simulink model "halfband"  (Simulink 6.6)
settings: Solver=VariableStepDiscrete  SolverMode=SingleTasking  StartTime=0.0  StopTime=32768/12.8e6  RelTol=1e-3
PreLoadFcn:
  | BandStop = [-3.42958342739925E-03
  | -3.96924972816777E-03
  | 3.36240242079605E-03
  | -3.69559301938797E-04
  | -1.05894149003527E-03
  | -8.14840987107909E-04
  | 1.7530676387556E-03
  | 1.34036064966413E-04
  | -1.14308266128403E-03
  | -9.49174097090283E-05
  | 6.03248952668495E-04
  | -1.37880491661181E-05
  | 3.01496212854443E-04
  | -1.51170938115043E-04
  | -1.36598686838681E-03
  | 5.70111740975978E-04
  | 2.54687450879208E-03
  | -1.30938351650158E-03
  | -3.70345932594267E-03
  | 2.34958094527142E-03
  | 4.70638508861354E-03
  | -3.63447325770534E-03
  | -5.42048880850211E-03
  | 5.04733658994141E-03
  | 5.73664963492967E-03
  | -6.41806248410625E-03
  | -5.59266496429819E-03
  | 7.54327536806022E-03
  | 4.98552853346454E-03
  | -8.19477711532235E-03
  | -0.003981934398949
  | 8.15112472755439E-03
  | 2.73310679605007E-03
  | -7.2335178325926E-03
  | -1.46109700227312E-03
  | 5.31968276105546E-03
  | 4.53554392900545E-04
  | -2.3624905104136E-03
  | -6.91383416719793E-06
  | -1.55028072571844E-03
  | 4.39442000874746E-04
  | 6.24871824720405E-03
  | -2.02046112670604E-03
  | -1.14453241392008E-02
  | 4.95112589832473E-03
  | 1.67661124768428E-02
  | -9.32507740199684E-03
  | -0.021782122503324
  | 1.51131098154502E-02
  | 2.60432898181234E-02
  | -2.21466012963762E-02
  | -2.91212142686167E-02
  | 3.01168095402658E-02
  | 3.06633074260529E-02
  | -3.86045681695146E-02
  | -3.04226536102195E-02
  | 4.71064979395918E-02
  | 2.82864592477587E-02
  | -0.055072115030369
  | -2.43008385443716E-02
  | 6.19536218373718E-02
  | 1.86731297334143E-02
  | -6.72663181480251E-02
  | -1.17570405164474E-02
  | 7.06188933644473E-02
  | 4.01415550094957E-03
  | 0.928234958756191
  | 4.01415550094957E-03
  | 7.06188933644473E-02
  | -1.17570405164474E-02
  | -6.72663181480251E-02
  | 1.86731297334143E-02
  | 6.19536218373718E-02
  | -2.43008385443716E-02
  | -0.055072115030369
  | 2.82864592477587E-02
  | 4.71064979395918E-02
  | -3.04226536102195E-02
  | -3.86045681695146E-02
  | 3.06633074260529E-02
  | 3.01168095402658E-02
  | -2.91212142686167E-02
  | -2.21466012963762E-02
  | 2.60432898181234E-02
  | 1.51131098154502E-02
  | -0.021782122503324
  | -9.32507740199684E-03
  | 1.67661124768428E-02
  | 4.95112589832473E-03
  | -1.14453241392008E-02
  | -2.02046112670604E-03
  | 6.24871824720405E-03
  | 4.39442000874746E-04
  | -1.55028072571844E-03
  | -6.91383416719793E-06
  | -2.3624905104136E-03
  | 4.53554392900545E-04
  | 5.31968276105546E-03
  | -1.46109700227312E-03
  | -7.2335178325926E-03
  | 2.73310679605007E-03
  | 8.15112472755439E-03
  | -0.003981934398949
  | -8.19477711532235E-03
  | 4.98552853346454E-03
  | 7.54327536806022E-03
  | -5.59266496429819E-03
  | -6.41806248410625E-03
  | 5.73664963492967E-03
  | 5.04733658994141E-03
  | -5.42048880850211E-03
  | -3.63447325770534E-03
  | 4.70638508861354E-03
  | 2.34958094527142E-03
  | -3.70345932594267E-03
  | -1.30938351650158E-03
  | 2.54687450879208E-03
  | 5.70111740975978E-04
  | -1.36598686838681E-03
  | -1.51170938115043E-04
  | 3.01496212854443E-04
  | -1.37880491661181E-05
  | 6.03248952668495E-04
  | -9.49174097090283E-05
  | -1.14308266128403E-03
  | 1.34036064966413E-04
  | 1.7530676387556E-03
  | -8.14840987107909E-04
  | -1.05894149003527E-03
  | -3.69559301938797E-04
  | 3.36240242079605E-03
  | -3.96924972816777E-03
  | -3.42958342739925E-03];
undefined symbols (not defined in the file): dfilt
libraries: xbsIndex_r4 x78, dsparch4 x3, dspsigops x2
(part 1 of 2)
settings Model: Creator=lcrockett  LastModifiedBy=Administrator
settings DataIOCC: SignalLoggingName=sigsOut
settings OptimizationCC: InlineParams=on
settings DebuggingCC: SignalResolutionControl=TryResolveAllWithWarning  SolverPrmCheckMsg=none  MultiTaskDSMMsg=warning  MultiTaskCondExecSysMsg=none  StrictBusMsg=None
settings HardwareCC: TargetUnknown=on
settings RTWCC: IncludeERTFirstTime=on
settings GRTTargetCC: ModelReferenceCompliant=off  MatFileLogging=off

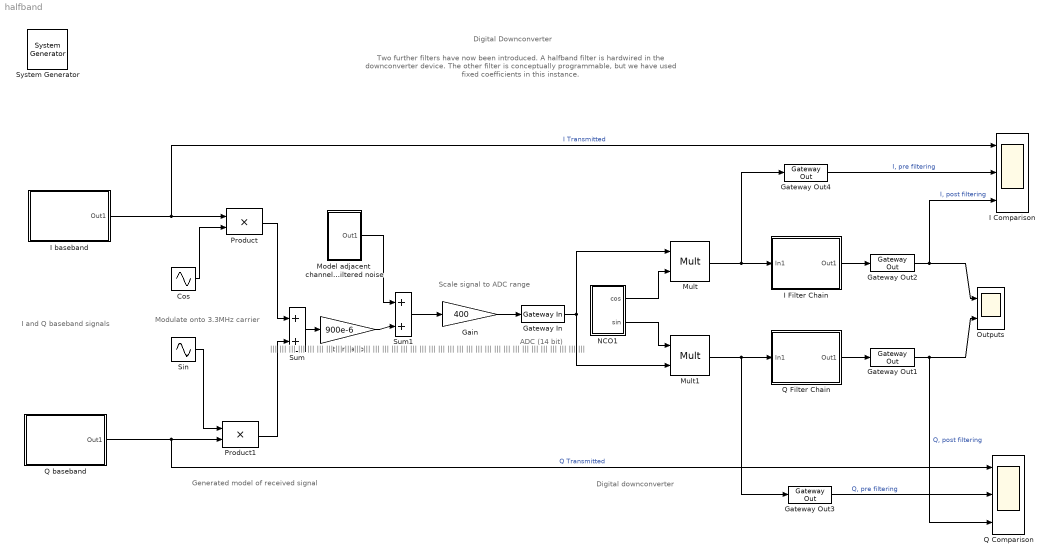
== system halfband ==
  note: Digital Downconverter
  note: Two further filters have now been introduced. A halfband filter is hardwired in the downconverter device.
      | The other filter is conceptually programmable, but we have used fixed coefficients in this instance.
  note: Digital downconverter
  note: ADC (14 bit)
  note: I and Q
      | baseband
      | signals
  note: Modulate onto
      | 3.3MHz carrier
  note: |||
      | |||
      | |||
      | |||
      | |||
      | |||
      | |||
      | |||
      | |||
      | |||
      | |||
      | |||
      | |||
      | |||
      | |||
      | |||
      | |||
      | |||
      | |||
      | |||
      | |||
      | |||
      | |||
      | |||
      | |||
      | |||
      | |||
      | |||
      | |||
      | |||
      | |||
      | |||
      | |||
      | |||
  note: Generated model of received signal
  note: Scale signal
      | to ADC range
  " System Generator" : xbsIndex_r4/ System Generator  Tag=genX  SystemSampleTime=-1  xilinxfamily=virtex2p  part=xc2vp30  speed=-7  package=ff896  synthesis_tool=XST  clock_wrapper=Clock Enables  directory=./netlist_05  testbench=off  simulink_period=1/12.8e6  sysclk_period=78.125  dcm_input_clock_period=100  incr_netlist=off  trim_vbits=Everywhere in SubSystem  dbl_ovrd=According to Block Masks  core_generation=According to Block Masks  run_coregen=off  deprecated_control=off  eval_field=0  block_type=sysgen
      settings: block_version=9.2.01
  Attenuation : Gain  Gain=900e-6  SaturateOnIntegerOverflow=on
  Cos : Sin  Frequency=2*pi*3.30999970436096e6  Phase=pi/2  SampleTime=1/12.8e6
  Gain : Gain  Gain=400  SaturateOnIntegerOverflow=on
  Gateway In : xbsIndex_r4/Gateway In  arith_type="Signed  (2's comp)"  n_bits=14  bin_pt=13  quantization="Round  (unbiased: +/- Inf)"  overflow=Saturate  period=1/12.8e6  dbl_ovrd=off  timing_constraint=None  locs_specified=off  LOCs={}  block_type=gatewayin
      settings: infoedit="Gateway in block.  Converts inputs of type Simulink integer, double and fixed point to  Xilinx fixed point type.<P><P>Hardware notes:  In hardware these blocks become top level input ports."  xl_area=[0, 0, 0, 0, 0, 0, 0]  block_version=VER_STRING_GOES_HERE
  Gateway Out{1..4} (4 alike) : xbsIndex_r4/Gateway Out  hdl_port=on  timing_constraint=None  locs_specified=off  LOCs={}  block_type=gatewayout
      settings: infoedit="Gateway out block.  Converts Xilinx fixed point inputs into ouputs of type Simulink integer, double, or fixed point.<P><P>Hardware notes:  In hardware these blocks become top level output ports or are discarded, depending on how they are configured."  xl_area=[0, 0, 0, 0, 0, 0, 0]  block_version=VER_STRING_GOES_HERE
  I Comparison : Scope  NumInputPorts=3
      settings: TimeRange=0.003  YMin=-2~-1~-0.4  YMax=2~1~0.4  DataFormat=Structure  MaxDataPoints=32768
  I Filter Chain : Subsystem
  I baseband : Subsystem
  Model adjacent  channels with  filtered noise : Subsystem
  Mult : xbsIndex_r4/Mult  precision=User Defined  arith_type="Signed  (2's comp)"  n_bits=15  bin_pt=14  quantization=Truncate  overflow=Wrap  en=off  latency=3  dbl_ovrd=off  use_behavioral_HDL=off  use_embedded=on  opt=Speed  optimum_pipeline=off  pipeline=on  use_rpm=on  placement_style=Rectangular shape  block_type=mult
      settings: infoedit=Hardware notes: To use the internal pipeline stage of the dedicated multiplier you must select 'Pipeline for maximum performance'.  xl_area=[0, 0, 0, 0, 0, 0, 0]  block_version=VER_STRING_GOES_HERE
  Mult1 : xbsIndex_r4/Mult  precision=User Defined  arith_type="Signed  (2's comp)"  n_bits=15  bin_pt=14  quantization=Truncate  overflow=Wrap  en=off  latency=3  dbl_ovrd=off  use_behavioral_HDL=off  use_embedded=on  opt=Speed  optimum_pipeline=off  pipeline=on  use_rpm=on  placement_style=Rectangular shape  block_type=mult
      settings: infoedit=Hardware notes: To use the internal pipeline stage of the dedicated multiplier you must select 'Pipeline for maximum performance'.  xl_area=[0, 0, 0, 0, 0, 0, 0]  block_version=VER_STRING_GOES_HERE
  NCO1 : Subsystem
  Outputs : Scope  NumInputPorts=2
      settings: TimeRange=0.003  YMin=-0.4~-0.4  YMax=0.4~0.4  SaveName=ScopeData2  DataFormat=Structure  MaxDataPoints=32768
  Product : Product  SaturateOnIntegerOverflow=on
  Product1 : Product  SaturateOnIntegerOverflow=on
  Q Comparison : Scope  NumInputPorts=3
      settings: TimeRange=0.003  YMin=-2~-1~-0.4  YMax=2~1~0.4  SaveName=ScopeData6  DataFormat=Structure  MaxDataPoints=32768
  Q Filter Chain : Subsystem
  Q baseband : Subsystem
  Sin : Sin  Frequency=2*pi*3.30999970436096e6  SampleTime=1/12.8e6
  Sum : Sum  Inputs=|++  SaturateOnIntegerOverflow=on
  Sum1 : Sum  Inputs=|++  SaturateOnIntegerOverflow=on
  wires:
  Gateway In/1 -> Mult/1, Mult1/2
  NCO1/2(sin) -> Mult1/1
  NCO1/1(cos) -> Mult/2
  Gateway Out1/1 -> Outputs/2, Q Comparison/3  "Q, post filtering"
  Gateway Out2/1 -> Outputs/1, I Comparison/3  "I, post filtering"
  Mult/1 -> I Filter Chain/1(In1), Gateway Out4/1
  Mult1/1 -> Gateway Out3/1, Q Filter Chain/1(In1)
  Gateway Out3/1 -> Q Comparison/2  "Q, pre filtering"
  I Filter Chain/1(Out1) -> Gateway Out2/1
  Q Filter Chain/1(Out1) -> Gateway Out1/1
  Gateway Out4/1 -> I Comparison/2  "I, pre filtering"
  I baseband/1(Out1) -> Product/1, I Comparison/1  "I Transmitted"
  Q baseband/1(Out1) -> Product1/2, Q Comparison/1  "Q Transmitted"
  Product/1 -> Sum/1
  Product1/1 -> Sum/2
  Sum/1 -> Attenuation/1
  Attenuation/1 -> Sum1/2
  Model adjacent  channels with  filtered noise/1(Out1) -> Sum1/1
  Sum1/1 -> Gain/1
  Sin/1 -> Product1/1
  Cos/1 -> Product/2
  Gain/1 -> Gateway In/1

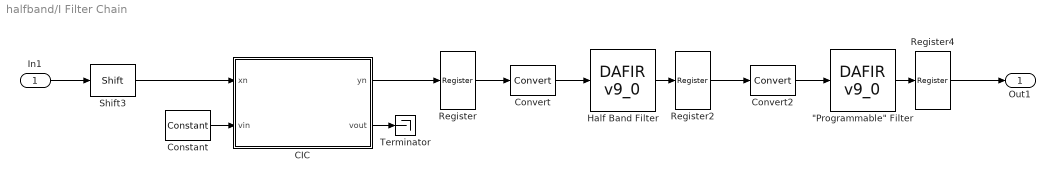
== system halfband/I Filter Chain ==
  In1 : Inport
  "\"Programmable\" Filter" : xbsIndex_r4/DAFIR v9_0   coef=[6.10352e-005 0.000793457 -0.000305176 -0.00518799 -0.00253296 0.0162964 0.0179443 -0.0342712 -0.0702209 0.0523071 0.303986 0.439972 0.303986 0.0523071 -0.0702209 -0.0342712 0.0179443 0.0162964 -0.00253296 -0.00518799 -0.000305176 0.000793457 6.10352e-005]  structure=Inferred from Coefficients  coef_n_bits=22  coef_bin_pt=21  over_sample=1  reload=off  valids=off  rst=off  latency=1  num_channels=1  serial_input=off  polyphase_behavior="Decimate:  2:1 (samples in:out)"  dbl_ovrd=off  explicit_period=off  period=1  use_isim=0  block_type=fir
      settings: infoedit="Hardware notes: Implemented using distributed arithmetic (DA).  The hardware over sampling rate determines the degree of parallelism.  A rate of one produces a fully parallel DA filter.  A rate of n (resp., n+1) for an n-bit input signal produces a fully serial implementation for a non-symmetric (resp., symmetric) impulse response.  Intermediate values produce implementations with intermediate levels of parallelism."  xl_area=[0, 0, 0, 0, 0, 0, 0]  block_version=VER_STRING_GOES_HERE
  CIC : Subsystem  mask{input_bitwidth=32, input_binpt=31, filter_type=Decimator, samp_rate_change=16, stages=5, differential_delay=1, latency=1}
      mask prompts: input_bitwidth "Input Bit Width"; input_binpt "Input Binary Point"; filter_type "Filter Type"; samp_rate_change "Sample Rate Change"; stages "Number of Stages"; differential_delay "Differential Delay"
      mask init:
      | [bg,fg] = xlcmap('XBlock',0);
      | iPos = get_param(gcb,'Position');
      | iWidth=iPos(3)-iPos(1); iHeight=iPos(4)-iPos(2);
      | iCx=iWidth/2;
      | iCy=iHeight/2;
      | [logoX, logoY] = xlogo(iPos);
      | % Print label on the block
      | if(filter_type == 2)
      |    str = sprintf('%d-Stage\n CIC\n%d:1 Decimator',stages, samp_rate_change);
      | else
      |    str = sprintf('%d-Stage\n CIC\n1:%d Interpolator',stages, samp_rate_change);	
      | end
      | cic_blk = [gcb '/CIC Filter'];
      | 
      | switch filter_type
      |     case 1
      |         set_param(cic_blk, 'filter_type','Interpolator');
      |     otherwise
      |         set_param(cic_blk, 'filter_type','Decimator');
      | end
      | 
      | set_param(cic_blk, 'm',num2str(differential_delay));
      settings: CopyFcn=set_param(gcb, 'LinkStatus', 'none');
      mask StyleString: edit,edit,popup(Interpolator|Decimator),edit,edit,popup(1|2|3|4),edit
      mask Display:
      | patch([0 iWidth iWidth 0],[0 0 iHeight iHeight] , bg);
      | patch(logoX,logoY , fg);
      | plot([0 0 iWidth iWidth 0], [0 iHeight iHeight 0 0]);
      | disp(str);
      | 
      | port_label('input',1,'xn');
      | port_label('input',2,'vin');
      | 
      | port_label('output',1,'yn');
      | port_label('output',2,'vout');
  Constant : xbsIndex_r4/Constant  arith_type=Boolean  const=1  n_bits=32  bin_pt=0  explicit_period=on  period=1/12.8e6  equ=P=C  opselect=C  inp2=PCIN>>17  opr=+  inp1=P  carry=CIN  dbl_ovrd=off  block_type=constant
      settings: block_version=VER_STRING_GOES_HERE
  Convert : xbsIndex_r4/Convert  arith_type="Signed  (2's comp)"  n_bits=24  bin_pt=23  quantization="Round  (unbiased: +/- Inf)"  overflow=Saturate  latency=0  dbl_ovrd=off  pipeline=off  block_type=convert
      settings: xl_area=[0, 0, 0, 0, 0, 0, 0]  block_version=VER_STRING_GOES_HERE
  Convert2 : xbsIndex_r4/Convert  arith_type="Signed  (2's comp)"  n_bits=24  bin_pt=23  quantization="Round  (unbiased: +/- Inf)"  overflow=Saturate  latency=0  dbl_ovrd=off  pipeline=off  block_type=convert
      settings: xl_area=[0, 0, 0, 0, 0, 0, 0]  block_version=VER_STRING_GOES_HERE
  Half Band Filter : xbsIndex_r4/DAFIR v9_0   coef=[ -0.000347137 0 0.00251317 0 -0.010158539 0 0.03055191 0 -0.081981659 0 0.309417725 0.5 0.309417725 0 -0.081981659 0 0.03055191 0 -0.010158539 0 0.00251317 0 -0.000347137]  structure=Half-Band Filter  coef_n_bits=24  coef_bin_pt=23  over_sample=1  reload=off  valids=off  rst=off  latency=1  num_channels=1  serial_input=off  polyphase_behavior="Decimate:  2:1 (samples in:out)"  dbl_ovrd=off  explicit_period=off  period=1  use_isim=0  block_type=fir
      settings: infoedit="Hardware notes: Implemented using distributed arithmetic (DA).  The hardware over sampling rate determines the degree of parallelism.  A rate of one produces a fully parallel DA filter.  A rate of n (resp., n+1) for an n-bit input signal produces a fully serial implementation for a non-symmetric (resp., symmetric) impulse response.  Intermediate values produce implementations with intermediate levels of parallelism."  xl_area=[0, 0, 0, 0, 0, 0, 0]  block_version=VER_STRING_GOES_HERE
  Register : xbsIndex_r4/Register  init=0  rst=off  en=off  dbl_ovrd=off  block_type=register
      settings: block_version=9.2.01
  Register2 : xbsIndex_r4/Register  init=0  rst=off  en=off  dbl_ovrd=off  block_type=register
      settings: block_version=9.2.01
  Register4 : xbsIndex_r4/Register  init=0  rst=off  en=off  dbl_ovrd=off  block_type=register
      settings: block_version=9.2.01
  Shift3 : xbsIndex_r4/Shift  shift_dir=Right  shift_bits=20  en=off  latency=0  precision=User Defined  arith_type="Signed  (2's comp)"  n_bits=32  bin_pt=31  quantization="Round  (unbiased: +/- Inf)"  overflow=Flag as error  dbl_ovrd=off  block_type=shift
      settings: xl_area=[0, 0, 0, 0, 0, 0, 0]  block_version=VER_STRING_GOES_HERE
  Terminator : Terminator
  Out1 : Outport
  wires:
  CIC/1(yn) -> Register/1
  CIC/2(vout) -> Terminator/1
  Half Band Filter/1 -> Register2/1
  "\"Programmable\" Filter"/1 -> Register4/1
  Convert/1 -> Half Band Filter/1
  Convert2/1 -> "\"Programmable\" Filter"/1
  Register/1 -> Convert/1
  Register2/1 -> Convert2/1
  In1/1 -> Shift3/1
  Register4/1 -> Out1/1
  Constant/1 -> CIC/2(vin)
  Shift3/1 -> CIC/1(xn)

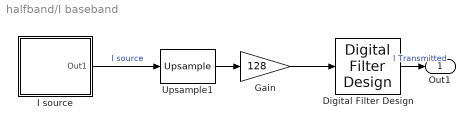
== system halfband/I baseband ==
  Digital Filter Design : dsparch4/Digital Filter Design  SystemSampleTime=-1  mwdsp_browser_bugfix_var=off
  Gain : Gain  Gain=128
  I source : Subsystem
  Upsample1 : dspsigops/Upsample  N=128  phase=0  ic=0  mode=Maintain input frame size
  Out1 : Outport
  wires:
  I source/1(Out1) -> Upsample1/1  "I source"
  Upsample1/1 -> Gain/1
  Gain/1 -> Digital Filter Design/1
  Digital Filter Design/1 -> Out1/1  "I Transmitted"

== system halfband/Model adjacent  channels with  filtered noise ==
  Digital Filter : dsparch4/Digital Filter  DialogController=dspdialog.DigitalFilter  DialogControllerArgs=DataTag2  TypePopup=FIR (all zeros)  IIRFiltStruct=Direct form II transposed  AllPoleFiltStruct=Direct form  FIRFiltStruct=Direct form  CoeffSource=Specify via dialog  NumCoeffs=[0.07 0.06 0.05 0.04 0.05 0.06 0.07]  DenCoeffs=[1]  BiQuadCoeffs=[1 0.3 0.4 1 0.1 0.2]  LatticeCoeffs=[0.2 0.4]  denIgnore=on  FiltPerSampPopup=One filter per frame  IC=0  ICnum=0  ICden=0  roundingMode=Floor  overflowMode=off  ScaleValues=1  scaleValueFracLength=14  stageInFracLength=15  stageOutFracLength=15  FilterSource=Specify via dialog  dfiltObjectName=dfilt.dffir([1 2 1])
  Random Number : RandomNumber  Variance=3.4e-7  Seed=1  SampleTime=1/12.8e6
  Out1 : Outport
  wires:
  Random Number/1 -> Digital Filter/1
  Digital Filter/1 -> Out1/1

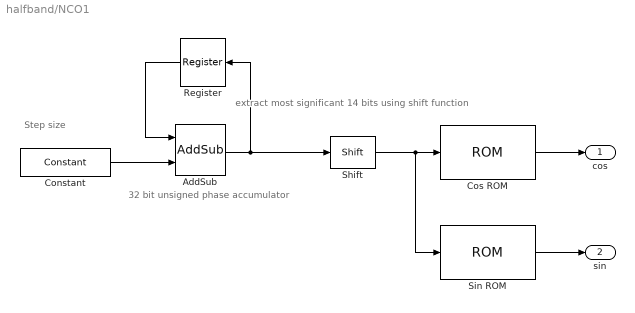
== system halfband/NCO1 ==
  note: extract most
      | significant
      | 14 bits using
      | shift function
  note: 32 bit unsigned phase accumulator
  note: Step size
  AddSub : xbsIndex_r4/AddSub  mode=Addition  use_carryin=off  use_carryout=off  en=off  latency=0  precision=User Defined  arith_type=Unsigned  n_bits=32  bin_pt=0  quantization=Truncate  overflow=Wrap  dbl_ovrd=off  use_behavioral_HDL=on  pipelined=off  use_rpm=on  block_type=addsub
      settings: xl_area=[0, 0, 0, 0, 0, 0, 0]  block_version=VER_STRING_GOES_HERE
  Constant : xbsIndex_r4/Constant  arith_type=Unsigned  const=1.11065e9  n_bits=32  bin_pt=0  explicit_period=on  period=1/12.8e6  equ=P=C  opselect=C  inp2=PCIN>>17  opr=+  inp1=P  carry=CIN  dbl_ovrd=off  block_type=constant
      settings: block_version=VER_STRING_GOES_HERE
  Cos ROM : xbsIndex_r4/ROM  depth=16384  initVector=cos(pi*(0:16383)/8192)  distributed_mem=Block RAM  rst=off  init_reg=0  en=off  latency=1  arith_type="Signed  (2's comp)"  n_bits=14  bin_pt=13  dbl_ovrd=off  optimize=Area  use_rpm=off  block_type=sprom
      settings: xl_area=[0, 0, 0, 0, 0, 0, 0]  block_version=VER_STRING_GOES_HERE
  Register : xbsIndex_r4/Register  Orientation=left  init=0  rst=off  en=off  dbl_ovrd=off  block_type=register
      settings: xl_area=[0, 0, 0, 0, 0, 0, 0]  block_version=VER_STRING_GOES_HERE
  Shift : xbsIndex_r4/Shift  shift_dir=Right  shift_bits=18  en=off  latency=0  precision=User Defined  arith_type=Unsigned  n_bits=14  bin_pt=0  quantization=Truncate  overflow=Wrap  dbl_ovrd=off  block_type=shift
      settings: xl_area=[0, 0, 0, 0, 0, 0, 0]  block_version=VER_STRING_GOES_HERE
  Sin ROM : xbsIndex_r4/ROM  depth=16384  initVector=sin(pi*(0:16383)/8192)  distributed_mem=Block RAM  rst=off  init_reg=0  en=off  latency=1  arith_type="Signed  (2's comp)"  n_bits=14  bin_pt=13  dbl_ovrd=off  optimize=Area  use_rpm=off  block_type=sprom
      settings: xl_area=[0, 0, 0, 0, 0, 0, 0]  block_version=VER_STRING_GOES_HERE
  cos : Outport
  sin : Outport  Port=2
  wires:
  Constant/1 -> AddSub/2
  AddSub/1 -> Register/1, Shift/1
  Register/1 -> AddSub/1
  Sin ROM/1 -> sin/1
  Cos ROM/1 -> cos/1
  Shift/1 -> Cos ROM/1, Sin ROM/1

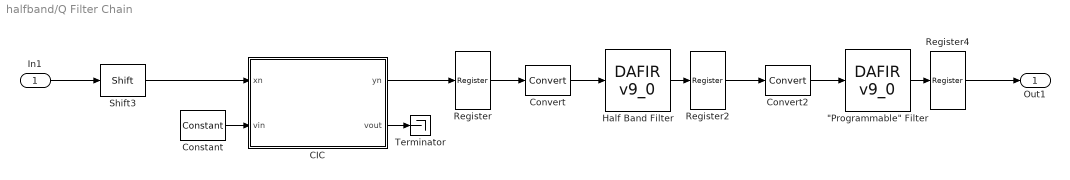
== system halfband/Q Filter Chain ==
  In1 : Inport
  "\"Programmable\" Filter" : xbsIndex_r4/DAFIR v9_0   coef=[6.10352e-005 0.000793457 -0.000305176 -0.00518799 -0.00253296 0.0162964 0.0179443 -0.0342712 -0.0702209 0.0523071 0.303986 0.439972 0.303986 0.0523071 -0.0702209 -0.0342712 0.0179443 0.0162964 -0.00253296 -0.00518799 -0.000305176 0.000793457 6.10352e-005]  structure=Inferred from Coefficients  coef_n_bits=22  coef_bin_pt=21  over_sample=1  reload=off  valids=off  rst=off  latency=1  num_channels=1  serial_input=off  polyphase_behavior="Decimate:  2:1 (samples in:out)"  dbl_ovrd=off  explicit_period=off  period=1  use_isim=0  block_type=fir
      settings: infoedit="Hardware notes: Implemented using distributed arithmetic (DA).  The hardware over sampling rate determines the degree of parallelism.  A rate of one produces a fully parallel DA filter.  A rate of n (resp., n+1) for an n-bit input signal produces a fully serial implementation for a non-symmetric (resp., symmetric) impulse response.  Intermediate values produce implementations with intermediate levels of parallelism."  xl_area=[0, 0, 0, 0, 0, 0, 0]  block_version=VER_STRING_GOES_HERE
  CIC : Subsystem  mask{input_bitwidth=32, input_binpt=31, filter_type=Decimator, samp_rate_change=16, stages=5, differential_delay=1, latency=1}
      mask prompts: input_bitwidth "Input Bit Width"; input_binpt "Input Binary Point"; filter_type "Filter Type"; samp_rate_change "Sample Rate Change"; stages "Number of Stages"; differential_delay "Differential Delay"
      mask init: same as halfband/I Filter Chain/CIC
      settings: CopyFcn=set_param(gcb, 'LinkStatus', 'none');
      mask StyleString: edit,edit,popup(Interpolator|Decimator),edit,edit,popup(1|2|3|4),edit
      mask Display:
      | patch([0 iWidth iWidth 0],[0 0 iHeight iHeight] , bg);
      | patch(logoX,logoY , fg);
      | plot([0 0 iWidth iWidth 0], [0 iHeight iHeight 0 0]);
      | disp(str);
      | 
      | port_label('input',1,'xn');
      | port_label('input',2,'vin');
      | 
      | port_label('output',1,'yn');
      | port_label('output',2,'vout');
  Constant : xbsIndex_r4/Constant  arith_type=Boolean  const=1  n_bits=32  bin_pt=0  explicit_period=on  period=1/12.8e6  equ=P=C  opselect=C  inp2=PCIN>>17  opr=+  inp1=P  carry=CIN  dbl_ovrd=off  block_type=constant
      settings: block_version=VER_STRING_GOES_HERE
  Convert : xbsIndex_r4/Convert  arith_type="Signed  (2's comp)"  n_bits=24  bin_pt=23  quantization="Round  (unbiased: +/- Inf)"  overflow=Saturate  latency=0  dbl_ovrd=off  pipeline=off  block_type=convert
      settings: xl_area=[0, 0, 0, 0, 0, 0, 0]  block_version=VER_STRING_GOES_HERE
  Convert2 : xbsIndex_r4/Convert  arith_type="Signed  (2's comp)"  n_bits=24  bin_pt=23  quantization="Round  (unbiased: +/- Inf)"  overflow=Saturate  latency=0  dbl_ovrd=off  pipeline=off  block_type=convert
      settings: xl_area=[0, 0, 0, 0, 0, 0, 0]  block_version=VER_STRING_GOES_HERE
  Half Band Filter : xbsIndex_r4/DAFIR v9_0   coef=[ -0.000347137 0 0.00251317 0 -0.010158539 0 0.03055191 0 -0.081981659 0 0.309417725 0.5 0.309417725 0 -0.081981659 0 0.03055191 0 -0.010158539 0 0.00251317 0 -0.000347137]  structure=Half-Band Filter  coef_n_bits=24  coef_bin_pt=23  over_sample=1  reload=off  valids=off  rst=off  latency=1  num_channels=1  serial_input=off  polyphase_behavior="Decimate:  2:1 (samples in:out)"  dbl_ovrd=off  explicit_period=off  period=1  use_isim=0  block_type=fir
      settings: infoedit="Hardware notes: Implemented using distributed arithmetic (DA).  The hardware over sampling rate determines the degree of parallelism.  A rate of one produces a fully parallel DA filter.  A rate of n (resp., n+1) for an n-bit input signal produces a fully serial implementation for a non-symmetric (resp., symmetric) impulse response.  Intermediate values produce implementations with intermediate levels of parallelism."  xl_area=[0, 0, 0, 0, 0, 0, 0]  block_version=VER_STRING_GOES_HERE
  Register : xbsIndex_r4/Register  init=0  rst=off  en=off  dbl_ovrd=off  block_type=register
      settings: block_version=9.2.01
  Register2 : xbsIndex_r4/Register  init=0  rst=off  en=off  dbl_ovrd=off  block_type=register
      settings: block_version=9.2.01
  Register4 : xbsIndex_r4/Register  init=0  rst=off  en=off  dbl_ovrd=off  block_type=register
      settings: block_version=9.2.01
  Shift3 : xbsIndex_r4/Shift  shift_dir=Right  shift_bits=20  en=off  latency=0  precision=User Defined  arith_type="Signed  (2's comp)"  n_bits=32  bin_pt=31  quantization="Round  (unbiased: +/- Inf)"  overflow=Flag as error  dbl_ovrd=off  block_type=shift
      settings: xl_area=[0, 0, 0, 0, 0, 0, 0]  block_version=VER_STRING_GOES_HERE
  Terminator : Terminator
  Out1 : Outport
  wires:
  CIC/1(yn) -> Register/1
  CIC/2(vout) -> Terminator/1
  Half Band Filter/1 -> Register2/1
  "\"Programmable\" Filter"/1 -> Register4/1
  Convert/1 -> Half Band Filter/1
  Convert2/1 -> "\"Programmable\" Filter"/1
  Register/1 -> Convert/1
  Register2/1 -> Convert2/1
  In1/1 -> Shift3/1
  Register4/1 -> Out1/1
  Constant/1 -> CIC/2(vin)
  Shift3/1 -> CIC/1(xn)

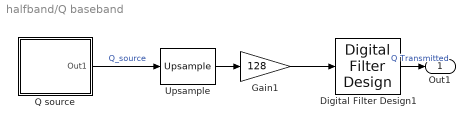
== system halfband/Q baseband ==
  Digital Filter Design1 : dsparch4/Digital Filter Design  SystemSampleTime=-1  mwdsp_browser_bugfix_var=off
  Gain1 : Gain  Gain=128
  Q source : Subsystem
  Upsample : dspsigops/Upsample  N=128  phase=0  ic=0  mode=Maintain input frame size
  Out1 : Outport
  wires:
  Q source/1(Out1) -> Upsample/1  "Q_source"
  Upsample/1 -> Gain1/1
  Gain1/1 -> Digital Filter Design1/1
  Digital Filter Design1/1 -> Out1/1  "Q Transmitted"

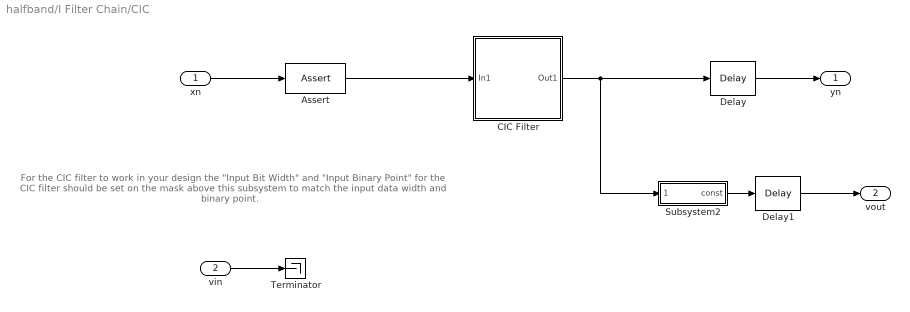
== system halfband/I Filter Chain/CIC ==
  note: For the CIC filter to work in your design
      |  the "Input Bit Width" and "Input Binary Point"
      | for the CIC filter should be set on the mask
      | above this subsystem to match the input data
      | width and binary point.
  xn : Inport
  vin : Inport  Port=2
  Assert : xbsIndex_r4/Assert  assert_type=on  type_source=Explicitly  arith_type="Signed  (2's comp)"  n_bits=input_bitwidth  bin_pt=input_binpt  assert_rate=off  rate_source=Explicitly  period=1  output_port=on  block_type=assert
      settings: infoedit=Asserts a user-defined sample rate and/or type on a signal.<P><P>Hardware notes: In hardware this block costs nothing.  block_version=VER_STRING_GOES_HERE
  CIC Filter : Subsystem  mask(CIC Filter){input_bitwidth=input_bitwidth, input_binpt=input_binpt, filter_type=Decimator, rate_change=samp_rate_change, stages=stages, m=1, pipeline=on, dbl_ovrd=off}
      mask prompts: input_bitwidth "Input Bit Width"; input_binpt "Input Binary Point"; filter_type "Filter Type"; rate_change "Sample Rate Change"; stages "Number of Stages"; m "Differential Delay"; pipeline "Pipeline Differentiators"; dbl_ovrd "Override with Doubles"
      mask help: Cascaded Integrated Comb (CIC) Filter
      mask init:
      | % CIC Single Channel v1.0
      | % Set Block Logo
      | [bg,fg] = xlcmap('XBlock',dbl_ovrd);
      | iPos = get_param(gcb,'Position');
      | iWidth=iPos(3)-iPos(1); iHeight=iPos(4)-iPos(2);
      | iCx=iWidth/2;
      | iCy=iHeight/2;
      | [logoX, logoY] = xlogo(iPos);	
      | 
      | % Print label on the block
      | if(filter_type == 2)
      |    str = sprintf('%d-Stage\n CIC\n%d:1 Decimator',stages, rate_change);
      | else
      |    str = sprintf('%d-Stage\n CIC\n1:%d Interpolator',stages, rate_change);	
      | end
      | 
      | set_param(gcb, 'LinkStatus', 'none');
      | sav_gcb=gcb;
      | 
      | % Make sure the entered values for stages and channels are positive integers
      | nstages = round(sum(abs(stages)));
      | 
      | % Calculate previous filter type 0 = Decimator, 1 = Interpolator
      | pft = find_system(sav_gcb, 'lookUnderMasks', 'all', 'FollowLinks','on','Name', 'Up Sample');
      | prev_filter_type = length(pft(:,1));
      | 
      | %calculate how many stages currently in the model
      | a = find_system(sav_gcb, 'lookUnderMasks', 'all', 'FollowLinks','on','masktype', 'Integrator Stage');
      | d = find_system(sav_gcb, 'lookUnderMasks', 'all', 'FollowLinks','on','masktype', 'Differentiator Stage');
      | prev_stages = length(a(:,1));
      | 
      | % issue an error if the number of stages entered is zero
      | if (nstages == 0)
      | 	nstages = prev_stages;
      | 	errordlg('Number of Stages must be more that zero')
      | end
      | 
      | if(filter_type == 2) % Decimator
      |    
      | 	
      |    if (prev_filter_type == 1) % was interpolator so turn to decimator
      | 	
      | 	  % disconnect all the wires from all the blocks
      |        for i= 2:prev_stages,
      | 	      delete_line(sav_gcb, ['Integrator' int2str(i-1) '/' int2str(1)], ['Integrator' int2str(i) '/' int2str(1)]);
      | 	      delete_line(sav_gcb, ['Differentiator' int2str(i-1) '/' int2str(1)], ['Differentiator' int2str(i) '/' int2str(1)]);
      |        end
      | 
      |        % disconnect the last blocks in the two sections
      |        delete_line(sav_gcb, ['Differentiator' int2str(prev_stages) '/' int2str(1)], ['Up Sample/1']);
      |        delete_line(sav_gcb, ['Integrator' int2str(prev_stages) '/' int2str(1)], 'Out1/1');
      | 	
      | 	   % delete the line from the Up sampler to the Integrator
      | 	   delete_line(sav_gcb, 'Up Sample/1', 'Integrator1/1'); 
      | 	   delete_line(sav_gcb, 'In1/1', 'Differentiator1/1'); 
      | 	   
      | 	   % Delete the Up Sampler and then replace with an Down Sampler
      | 	   pup = get_param([sav_gcb '/Up Sample'], 'position');
      | 	   delete_block([sav_gcb '/Up Sample']);
      | 	   load_system('xbsIndex_r4');
      | 	   add_block('xbsIndex_r4/Down Sample', [sav_gcb '/Down Sample'], 'sample_ratio', 'rate_change','sample_phase', 'First Value of Frame', 'position', [pup(1), pup(2), pup(3),pup(4)]);
      | 	   
      | 	   % Switch the Integrators and Decimators around
      | 	   for i=1:prev_stages,
      | 		   tempi = get_param([sav_gcb '/Integrator' int2str(i)], 'position');
      | 	       tempd = get_param([sav_gcb '/Differentiator' int2str(i)], 'position');
      | 		   set_param([sav_gcb '/Differentiator' int2str(i)], 'position', [tempi(1), tempi(2), tempi(3), tempi(4)], 'output_bitwidth', 'ceil(stages*log2(rate_change*m) + input_bitwidth)');
      | 		   set_param([sav_gcb '/Integrator' int2str(i)], 'position', [tempd(1), tempd(2), tempd(3), tempd(4)]);
      | 	   end
      | 	   	   	
      | 	   % add back in the lines
      |        add_line(sav_gcb, 'In1/1', 'Integrator1/1', 'autorouting', 'on');
      | 	   add_line(sav_gcb, ['Integrator' int2str(prev_stages) '/1'], 'Down Sample/1', 'autorouting', 'on');
      | 	   add_line(sav_gcb, 'Down Sample/1', 'Differentiator1/1', 'autorouting', 'on');
      | 	   add_line(sav_gcb, ['Differentiator' int2str(prev_stages) '/1'], 'Out1/1', 'autorouting', 'on');
      | 	   for i= 2:prev_stages,
      |           add_line(sav_gcb, ['Integrator' int2str(i-1) '/1'], ['Integrator' int2str(i) '/' int2str(1)], 'autorouting', 'on');
      |           add_line(sav_gcb, ['Differentiator' int2str(i-1) '/1'], ['Differentiator' int2str(i) '/' int2str(1)], 'autorouting', 'on');
      | 	   end
      | 		
      |        %Set the Output bit widths of Differentiator and Integrator stages
      |        set_param([sav_gcb '/Differentiator1'], 'output_bitwidth', 'ceil(stages*log2(rate_change*m) + input_bitwidth)');
      | 	   	   %Set the Output bit width of Integrator stages
      | 	   %Calculate the Interpolator Integrator Output Bit Growth
      |        for i= 1:nstages,
      | 			 j = nstages+i;
      | 	         set_param([sav_gcb '/Integrator' int2str(i)], 'output_bitwidth', 'ceil(stages*log2(rate_change*m) + input_bitwidth)');
      |              set_param([sav_gcb '/Differentiator' int2str(i)], 'output_bitwidth', 'ceil(stages*log2(rate_change*m) + input_bitwidth)');
      | 	   end
      | 	   
      |    end
      |    
      |    if (nstages ~= prev_stages)
      |     
      |        % disconnect all the wires from all the blocks
      |        for i= 2:prev_stages,
      | 	      delete_line(sav_gcb, ['Integrator' int2str(i-1) '/' int2str(1)], ['Integrator' int2str(i) '/' int2str(1)]);
      | 	      delete_line(sav_gcb, ['Differentiator' int2str(i-1) '/' int2str(1)], ['Differentiator' int2str(i) '/' int2str(1)]);
      |        end
      | 
      |        % disconnect the last blocks in the two sections
      |        delete_line(sav_gcb, ['Integrator' int2str(prev_stages) '/' int2str(1)], ['Down Sample/1']);
      |        delete_line(sav_gcb, ['Differentiator' int2str(prev_stages) '/' int2str(1)], 'Out1/1');
      | 	
      | 	   % delete the line from the down sampler to the differentiator
      | 	   delete_line(sav_gcb, 'Down Sample/1', 'Differentiator1/1');
      | 	
      | 	   % Remove all the blocks except the first one (as we always will have one)
      |        for i=2:prev_stages,
      | 		  delete_block([sav_gcb '/Differentiator' int2str(i)]);
      | 	      delete_block([sav_gcb '/Integrator' int2str(i)]);
      |        end
      | 	   
      | 	   %Set the Output bit width of Differentiator stages
      |        set_param([sav_gcb '/Differentiator1'], 'output_bitwidth', 'ceil(stages*log2(rate_change*m) + input_bitwidth)');
      | 	   
      | 	   % collect data on the position of existing blocks
      | 	   pi = get_param([sav_gcb '/Integrator1'], 'position');
      | 	   pd = get_param([sav_gcb '/Differentiator1'], 'position');
      | 	   set_param([sav_gcb '/Differentiator1'], 'position', [pi(1)+(nstages+1)*80, pd(2), pi(3)+(nstages+1)*80, pd(4)]);
      | 	   pd = get_param([sav_gcb '/Differentiator1'], 'position');
      | 	
      | 	   % move the current blocks to accomadate for new blocks to be added 
      | 	   pds = get_param([sav_gcb '/Down Sample'], 'position');
      | 	   set_param([sav_gcb '/Down Sample'], 'position', [pi(1)+(nstages)*80, pds(2), pi(3)+(nstages)*80, pds(4)]);
      | 	   
      | 	   po = get_param([sav_gcb '/Out1'], 'position');
      | 	   set_param([sav_gcb '/Out1'], 'position', [pd(1)+(nstages+1)*80, po(2), pd(1)+(po(3)-po(1))+(nstages+1)*80, po(4)]);	
      | 	
      | 	   % add back in the line between the Down Sampler and the 1st Differentiator
      |        add_line(sav_gcb, 'Down Sample/1', ['Differentiator1/' int2str(1)], 'autorouting', 'on');
      | 
      | 	   % Only add blocks if more than one stage is required
      | 	   if (nstages ~= 1)
      | 		
      | 	       % Add in a copy of the first block to make up the required number of stages
      |            for i=2:nstages,
      |                add_block([sav_gcb '/Integrator1'], [sav_gcb '/Integrator' int2str(i)], 'position', [pi(1)+(i-1)*80, pi(2), pi(3)+(i-1)*80, pi(4)]);
      | 		       add_block([sav_gcb '/Differentiator1'], [sav_gcb '/Differentiator' int2str(i)], 'position', [pd(1)+(i-1)*80, pd(2), pd(3)+(i-1)*80, pd(4)]);
      | 	       end
      | 		
      | 	       % Connect up the wires to each block use autorouting
      |            for i= 2:nstages,
      |  		       add_line(sav_gcb, ['Integrator' int2str(i-1) '/' int2str(1)], ['Integrator' int2str(i) '/' int2str(1)], 'autorouting', 'on');
      | 	           add_line(sav_gcb, ['Differentiator' int2str(i-1) '/' int2str(1)], ['Differentiator' int2str(i) '/' int2str(1)], 'autorouting', 'on');
      |            end
      | 	    end
      | 	       % Connect the last blocks in the two sections
      |            add_line(sav_gcb, ['Integrator' int2str(nstages) '/' int2str(1)], ['Down Sample/1'], 'autorouting', 'on');
      |            add_line(sav_gcb, ['Differentiator' int2str(nstages) '/' int2str(1)], ['Out1/1'], 'autorouting', 'on');
      |    end
      | 
      | else % Interpolator
      |    
      | 	
      | 	if (prev_filter_type == 0) % was decimator so turn to interpolator
      | 	
      | 	  % disconnect all the wires from all the blocks
      |        for i= 2:prev_stages,
      | 	      delete_line(sav_gcb, ['Integrator' int2str(i-1) '/' int2str(1)], ['Integrator' int2str(i) '/' int2str(1)]);
      | 	      delete_line(sav_gcb, ['Differentiator' int2str(i-1) '/' int2str(1)], ['Differentiator' int2str(i) '/' int2str(1)]);
      |        end
      | 
      |        % disconnect the last blocks in the two sections
      |        delete_line(sav_gcb, ['Integrator' int2str(prev_stages) '/' int2str(1)], ['Down Sample/1']);
      |        delete_line(sav_gcb, ['Differentiator' int2str(prev_stages) '/' int2str(1)], 'Out1/1');
      | 	
      | 	   % delete the line from the down sampler to the Differentiator
      | 	   delete_line(sav_gcb, 'Down Sample/1', 'Differentiator1/1'); 
      | 	   delete_line(sav_gcb, 'In1/1', 'Integrator1/1'); 
      | 	   
      | 	   % Delete the Down Sampler and then replace with a Up Sampler
      | 	   pdwn = get_param([sav_gcb '/Down Sample'], 'position');
      | 	   delete_block([sav_gcb '/Down Sample']);
      | 	   load_system('xbsIndex_r4');
      | 	   add_block('xbsIndex_r4/Up Sample', [sav_gcb '/Up Sample'], 'sample_ratio', 'rate_change', 'position', [pdwn(1), pdwn(2), pdwn(3), pdwn(4)]);
      | 	   
      | 	   % Switch the Integrators and Decimators around
      | 	   for i=1:prev_stages,
      | 		   tempi = get_param([sav_gcb '/Integrator' int2str(i)], 'position');
      | 	       tempd = get_param([sav_gcb '/Differentiator' int2str(i)], 'position');
      | 		   set_param([sav_gcb '/Differentiator' int2str(i)], 'position', [tempi(1), tempi(2), tempi(3), tempi(4)], 'output_bitwidth', [int2str(i) '+ input_bitwidth']);
      | 		   set_param([sav_gcb '/Integrator' int2str(i)], 'position', [tempd(1), tempd(2), tempd(3), tempd(4)]);
      | 	   end
      | 	   	   	
      | 	   % add back in the lines
      |        add_line(sav_gcb, 'In1/1', 'Differentiator1/1', 'autorouting', 'on');
      | 	   add_line(sav_gcb, ['Differentiator' int2str(prev_stages) '/1'], 'Up Sample/1', 'autorouting', 'on');
      | 	   add_line(sav_gcb, 'Up Sample/1', 'Integrator1/1', 'autorouting', 'on');
      | 	   add_line(sav_gcb, ['Integrator' int2str(prev_stages) '/1'], 'Out1/1', 'autorouting', 'on');
      | 	   for i= 2:prev_stages,
      |           add_line(sav_gcb, ['Integrator' int2str(i-1) '/1'], ['Integrator' int2str(i) '/1'], 'autorouting', 'on');
      |           add_line(sav_gcb, ['Differentiator' int2str(i-1) '/1'], ['Differentiator' int2str(i) '/1'], 'autorouting', 'on');
      | 	   end
      | 	   
      | 	   %Set the Output bit width of Integrator stages
      | 	   %Calculate the Interpolator Integrator Output Bit Growth
      |        for i= 1:nstages,
      | 			 j = nstages+i;
      | 	         set_param([sav_gcb '/Integrator' int2str(i)], 'output_bitwidth', ['ceil(log2(2^(2*stages-' int2str(j) ')*(rate_change*m)^(' int2str(j) '-stages)) + input_bitwidth)']);
      | 	   end
      | 		
      |    end
      |    
      | 	
      | 	if (nstages ~= prev_stages)
      |     
      |        % disconnect all the wires from all the blocks
      |        for i= 2:prev_stages,
      | 	      delete_line(sav_gcb, ['Integrator' int2str(i-1) '/' int2str(1)], ['Integrator' int2str(i) '/' int2str(1)]);
      | 	      delete_line(sav_gcb, ['Differentiator' int2str(i-1) '/' int2str(1)], ['Differentiator' int2str(i) '/' int2str(1)]);
      |        end
      | 
      |        % disconnect the last blocks in the two sections
      |        delete_line(sav_gcb, ['Differentiator' int2str(prev_stages) '/' int2str(1)], ['Up Sample/1']);
      |        delete_line(sav_gcb, ['Integrator' int2str(prev_stages) '/' int2str(1)], 'Out1/1');
      |        
      | 	
      | 	   % delete the line from the Up sampler to the Integrator1 for movement later
      | 	   delete_line(sav_gcb, 'Up Sample/1', 'Integrator1/1'); 
      | 	
      | 	   % Remove all the blocks except the first one (as we always will have one)
      |        for i=2:prev_stages,
      | 		  delete_block([sav_gcb '/Differentiator' int2str(i)]);
      | 	      delete_block([sav_gcb '/Integrator' int2str(i)]);
      |        end
      | 	
      | 	   %Set the Output bit width of first Differentiator stage (other are set as copies of this block)
      |        set_param([sav_gcb '/Differentiator1'], 'output_bitwidth', '1 + input_bitwidth');
      | 	   
      | 	   % collect data on the position of existing blocks
      | 	   pi = get_param([sav_gcb '/Integrator1'], 'position');
      | 	   pd = get_param([sav_gcb '/Differentiator1'], 'position');
      | 	   set_param([sav_gcb '/Integrator1'], 'position', [pd(1)+(nstages+1)*80, pi(2), pd(3)+(nstages+1)*80, pi(4)]);
      | 	   pi = get_param([sav_gcb '/Integrator1'], 'position');
      | 	
      | 	   % move the current blocks to accomadate for new blocks to be added 
      | 	   pus = get_param([sav_gcb '/Up Sample'], 'position');
      | 	   set_param([sav_gcb '/Up Sample'], 'position', [pd(1)+(nstages)*80, pus(2), pd(3)+(nstages)*80, pus(4)]);
      | 	
      | 	   po = get_param([sav_gcb '/Out1'], 'position');
      |        set_param([sav_gcb '/Out1'], 'position', [pi(1)+(nstages+1)*80, po(2), pi(1)+(po(3)-po(1))+(nstages+1)*80, po(4)]);	
      |       
      | 	
      | 	   % add back in the line between the Up Sampler and the 1st Integrator1
      | 	   add_line(sav_gcb, 'Up Sample/1', 'Integrator1/1', 'autorouting', 'on');
      | 	   
      | 	   % Only add blocks if more than one stage is required
      | 	   if (nstages ~= 1)
      | 		
      | 	       % Add in a copy of the first block to make up the required number of stages
      |            for i=2:nstages,
      |                add_block([sav_gcb '/Integrator1'], [sav_gcb '/Integrator' int2str(i)], 'position', [pi(1)+(i-1)*80, pi(2), pi(3)+(i-1)*80, pi(4)]);
      | 		       add_block([sav_gcb '/Differentiator1'], [sav_gcb '/Differentiator' int2str(i)], 'position', [pd(1)+(i-1)*80, pd(2), pd(3)+(i-1)*80, pd(4)], 'output_bitwidth', [int2str(i) '+ input_bitwidth']);
      | 	       end
      | 		
      | 	       % Connect up the wires to each block use autorouting
      |            for i= 2:nstages,
      |  		       add_line(sav_gcb, ['Integrator' int2str(i-1) '/' int2str(1)], ['Integrator' int2str(i) '/' int2str(1)], 'autorouting', 'on');
      | 	           add_line(sav_gcb, ['Differentiator' int2str(i-1) '/' int2str(1)], ['Differentiator' int2str(i) '/' int2str(1)], 'autorouting', 'on');
      |            end
      | 	    end
      | 	       % Connect the last blocks in the two sections
      |            add_line(sav_gcb, ['Differentiator' int2str(nstages) '/1'], ['Up Sample/1'], 'autorouting', 'on');
      |            add_line(sav_gcb, ['Integrator' int2str(nstages) '/1'], ['Out1/1'], 'autorouting', 'on');
      | 		   
      | 	     %Set the Output bit width of Integrator stages
      | 	     %Calculate the Interpolator Integrator Output Bit Growth
      |           for i= 1:nstages,
      | 			 j = nstages+i;
      | 	         set_param([sav_gcb '/Integrator' int2str(i)], 'output_bitwidth', ['ceil(log2(2^(2*stages-' int2str(j) ')*(rate_change*m)^(' int2str(j) '-stages)) + input_bitwidth)']);
      | 	      end
      |    end
      | 	  
      | end
      | 
      | 
      | % Set the pipelining to ON or OFF on the differentiators
      | if (pipeline == 0)
      | 	for i= 1:nstages
      | 		set_param([sav_gcb '/Differentiator' int2str(i), '/AddSub'], 'latency', '0')
      | 	end
      | else
      | 	for i= 1:nstages
      | 		set_param([sav_gcb '/Differentiator' int2str(i), '/AddSub'], 'latency' ,'1')
      | 	end
      | end
      | 
      | % Set the overide with doubles on with selected
      | % Find all the Xilinx Blocks in the system
      | total = find_system(sav_gcb, 'lookUnderMasks', 'all', 'FollowLinks','on','Blocktype', 'S-Function');
      | total_length = length(total(:,1));
      | 
      | if (dbl_ovrd == 0)
      | 	for i= 1:total_length,
      |     	set_param(char(total(i)), 'dbl_ovrd', 'off');
      | 	end
      | else
      | 	for i= 1:total_length,
      | 		set_param(char(total(i)), 'dbl_ovrd', 'on');
      | 	end
      | 	[bg,fg]=xlcmap('XBlock',1);
      | end
      settings: CopyFcn=set_param(gcb, 'LinkStatus', 'none');
      mask Help: eval('xlWeb(xlhtmldoclink(''CIC Filter''))');
      mask StyleString: edit,edit,popup(Interpolator|Decimator),edit,edit,popup(1|2|3|4),checkbox,checkbox
      mask Display:
      | patch([0 iWidth iWidth 0],[0 0 iHeight iHeight] , bg);
      | patch(logoX,logoY , fg);
      | plot([0 0 iWidth iWidth 0], [0 iHeight iHeight 0 0]);
      | disp(str)
  Delay : xbsIndex_r4/Delay  en=off  latency=latency-1  dbl_ovrd=off  reg_retiming=off  block_type=delay
      settings: infoedit=Hardware notes: A delay line is a chain, each link of which is an SRL16 followed by a flip-flop. If register retiming is enabled, the delay line is a chain of flip-flops.  block_version=VER_STRING_GOES_HERE
  Delay1 : xbsIndex_r4/Delay  en=off  latency=latency  dbl_ovrd=off  reg_retiming=off  block_type=delay
      settings: infoedit=Hardware notes: A delay line is a chain, each link of which is an SRL16 followed by a flip-flop. If register retiming is enabled, the delay line is a chain of flip-flops.  block_version=VER_STRING_GOES_HERE
  Subsystem2 : Subsystem
  Terminator : Terminator
  yn : Outport
  vout : Outport  Port=2
  wires:
  Assert/1 -> CIC Filter/1(In1)
  Subsystem2/1(const) -> Delay1/1
  vin/1 -> Terminator/1
  xn/1 -> Assert/1
  CIC Filter/1(Out1) -> Subsystem2/1(sample), Delay/1
  Delay/1 -> yn/1
  Delay1/1 -> vout/1

== system halfband/I baseband/I source ==
  Random Number2 : RandomNumber  Seed=777  SampleTime=1/100e3
  Sign2 : Signum
  Out1 : Outport
  wires:
  Random Number2/1 -> Sign2/1
  Sign2/1 -> Out1/1
